simulink model "airTrackHangingMass"  (R2021a)
settings: Solver=VariableStepAuto  StartTime=0.0  StopTime=30  FixedStep=0.02  MaxStep=0.002  RelTol=1e-6  EnableMultiTasking=on
PostLoadFcn:
  | disp('default settings')
  | 
  | % Default starting positions
  | x0_cart1 = -0.2
  | x0_cart2 = 0.8
  | x0_gate1 = -0.4
  | x0_gate2 = 0.4
  | 
  | % How much damping the carts feel
  | dampingCoef = 0.01 % N/(m/s)
  | 
  | % Hanger damping
  | pulleyDamping = 0;
  | 
  | % Max measurement noise for the gates
  | noise_max = 0.01 % seconds
  | 
  | % How many time steps to show in the history
  | nHistory = 4
  | 
  | % Based on the provided STLs
  | cart_length = 0.15
  | 
  | subsystems = find_system(gcs,'BlockType','SubSystem');
  | p = Simulink.Mask.get(subsystems{1});
  | p.Parameters(1).Value = '-0.8';
  | p.Parameters(2).Value = '0';
  | p.Parameters(3).Value = '-0.4';
  | p.Parameters(4).Value = '0.4';
  | p.Parameters(5).Value = '0';
  | p.Parameters(6).Value = '0';
  | p.Parameters(7).Value = '20';
undefined symbols (not defined in the file): Push, X, x, Y, Z
libraries: sm_lib x73, simulink x12, nesl_utility x7
(part 3 of 3)

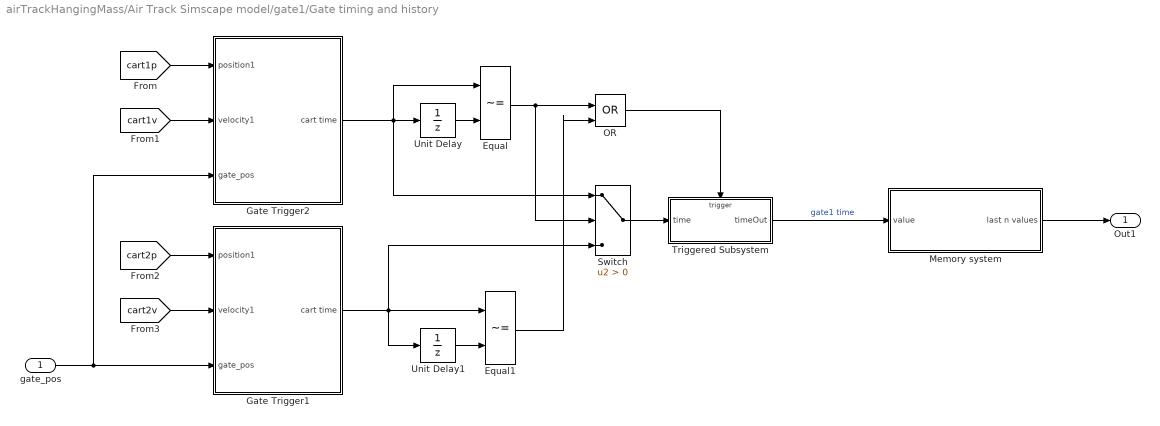
== system airTrackHangingMass/Air Track Simscape model/gate1/Gate timing and history ==
  gate_pos : Inport
  Equal : RelationalOperator  Operator=~=  OutDataTypeStr=boolean  RndMeth=Simplest
  Equal1 : RelationalOperator  Operator=~=  OutDataTypeStr=boolean  RndMeth=Simplest
  Gate Trigger1 : Subsystem
  Gate Trigger2 : Subsystem
  Memory system : Subsystem
  OR : Logic  Operator=OR  IconShape=distinctive  AllPortsSameDT=off  OutDataTypeStr=boolean
  Switch : Switch  Criteria=u2 > Threshold
  Triggered Subsystem : Subsystem  TreatAsAtomicUnit=on
  Unit Delay : UnitDelay  SampleTime=-1  HasFrameUpgradeWarning=on
  Unit Delay1 : UnitDelay  SampleTime=-1  HasFrameUpgradeWarning=on
  Out1 : Outport
  wires:
  Gate Trigger1/1(cart time) -> Switch/3, Equal1/1, Unit Delay1/1
  gate_pos/1 -> Gate Trigger2/3(gate_pos), Gate Trigger1/3(gate_pos)
  OR/1 -> Triggered Subsystem/Trigger
  [cart2p] -> Gate Trigger1/1(position1)
  Equal/1 -> Switch/2, OR/1
  [cart1v] -> Gate Trigger2/2(velocity1)
  Triggered Subsystem/1(timeOut) -> Memory system/1(value)  "gate1 time"
  [cart2v] -> Gate Trigger1/2(velocity1)
  Unit Delay/1 -> Equal/2
  Gate Trigger2/1(cart time) -> Switch/1, Equal/1, Unit Delay/1
  Equal1/1 -> OR/2
  Unit Delay1/1 -> Equal1/2
  [cart1p] -> Gate Trigger2/1(position1)
  Switch/1 -> Triggered Subsystem/1(time)
  Memory system/1(last n values) -> Out1/1

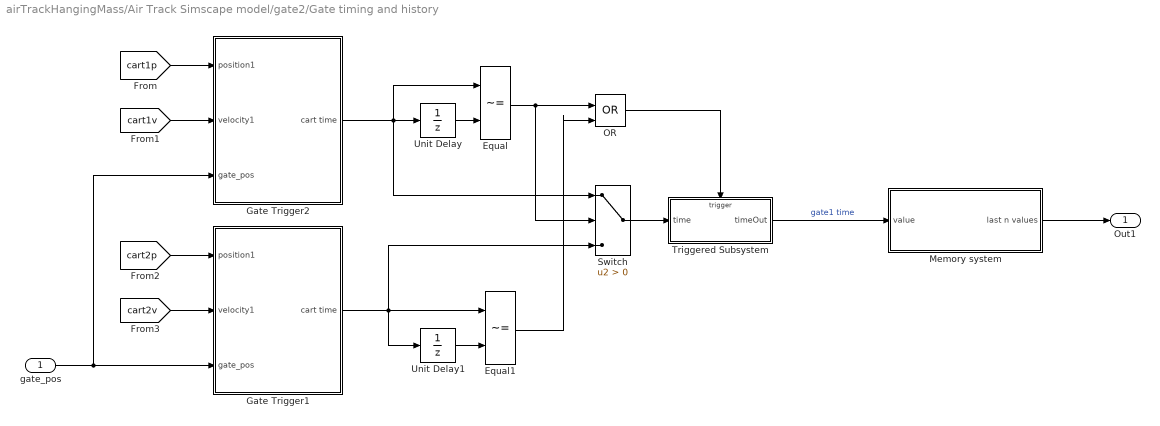
== system airTrackHangingMass/Air Track Simscape model/gate2/Gate timing and history ==
  gate_pos : Inport
  Equal : RelationalOperator  Operator=~=  OutDataTypeStr=boolean  RndMeth=Simplest
  Equal1 : RelationalOperator  Operator=~=  OutDataTypeStr=boolean  RndMeth=Simplest
  Gate Trigger1 : Subsystem
  Gate Trigger2 : Subsystem
  Memory system : Subsystem
  OR : Logic  Operator=OR  IconShape=distinctive  AllPortsSameDT=off  OutDataTypeStr=boolean
  Switch : Switch  Criteria=u2 > Threshold
  Triggered Subsystem : Subsystem  TreatAsAtomicUnit=on
  Unit Delay : UnitDelay  SampleTime=-1  HasFrameUpgradeWarning=on
  Unit Delay1 : UnitDelay  SampleTime=-1  HasFrameUpgradeWarning=on
  Out1 : Outport
  wires:
  Gate Trigger1/1(cart time) -> Switch/3, Equal1/1, Unit Delay1/1
  gate_pos/1 -> Gate Trigger2/3(gate_pos), Gate Trigger1/3(gate_pos)
  OR/1 -> Triggered Subsystem/Trigger
  [cart2p] -> Gate Trigger1/1(position1)
  Equal/1 -> Switch/2, OR/1
  [cart1v] -> Gate Trigger2/2(velocity1)
  Triggered Subsystem/1(timeOut) -> Memory system/1(value)  "gate1 time"
  [cart2v] -> Gate Trigger1/2(velocity1)
  Unit Delay/1 -> Equal/2
  Gate Trigger2/1(cart time) -> Switch/1, Equal/1, Unit Delay/1
  Equal1/1 -> OR/2
  Unit Delay1/1 -> Equal1/2
  [cart1p] -> Gate Trigger2/1(position1)
  Switch/1 -> Triggered Subsystem/1(time)
  Memory system/1(last n values) -> Out1/1

== system airTrackHangingMass/Air Track Simscape model/Cart1/short pulse/Triggered Subsystem ==
  In1 : Inport
  Trigger : TriggerPort  VariantControl=Variant
  Out1 : Outport
  wires:
  In1/1 -> Out1/1

== system airTrackHangingMass/Air Track Simscape model/Cart1/short pulse/Triggered Subsystem1 ==
  In1 : Inport
  Trigger : TriggerPort  VariantControl=Variant
  Out1 : Outport
  wires:
  In1/1 -> Out1/1

== system airTrackHangingMass/Air Track Simscape model/Cart2/short pulse2/Triggered Subsystem ==
  In1 : Inport
  Trigger : TriggerPort  VariantControl=Variant
  Out1 : Outport
  wires:
  In1/1 -> Out1/1

== system airTrackHangingMass/Air Track Simscape model/Cart2/short pulse2/Triggered Subsystem1 ==
  In1 : Inport
  Trigger : TriggerPort  VariantControl=Variant
  Out1 : Outport
  wires:
  In1/1 -> Out1/1

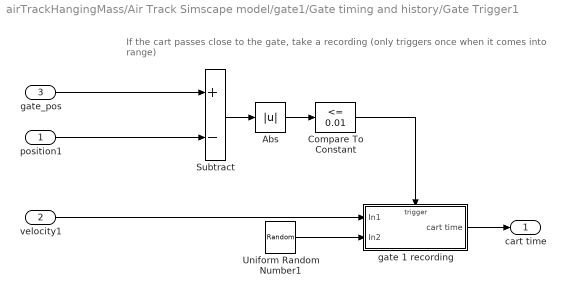
== system airTrackHangingMass/Air Track Simscape model/gate1/Gate timing and history/Gate Trigger1 ==
  note: If the cart passes close to the gate, take a recording
      | (only triggers once when it comes into range)
  position1 : Inport
  velocity1 : Inport  Port=2
  gate_pos : Inport  Port=3
  Abs : Abs
  Compare To Constant : simulink/Logic and Bit Operations/Compare To Constant  relop=<=  const=0.01  OutDataTypeStr=boolean
  Subtract : Sum  Inputs=+-
  Uniform Random Number1 : UniformRandomNumber  Minimum=-noise_max/2  Maximum=noise_max/2  SampleTime=0.1
  gate 1 recording : Subsystem  TreatAsAtomicUnit=on
  cart time : Outport
  wires:
  position1/1 -> Subtract/2
  velocity1/1 -> gate 1 recording/1(In1)
  gate 1 recording/1(cart time) -> cart time/1
  Abs/1 -> Compare To Constant/1
  Subtract/1 -> Abs/1
  Compare To Constant/1 -> gate 1 recording/Trigger
  Uniform Random Number1/1 -> gate 1 recording/2(In2)
  gate_pos/1 -> Subtract/1

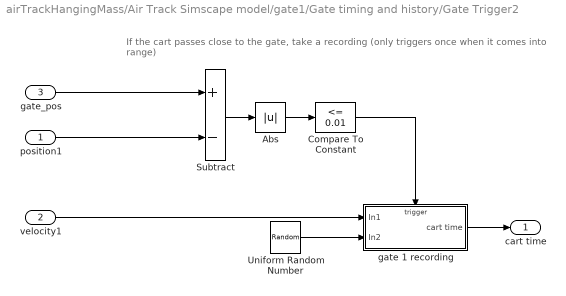
== system airTrackHangingMass/Air Track Simscape model/gate1/Gate timing and history/Gate Trigger2 ==
  note: If the cart passes close to the gate, take a recording
      | (only triggers once when it comes into range)
  position1 : Inport
  velocity1 : Inport  Port=2
  gate_pos : Inport  Port=3
  Abs : Abs
  Compare To Constant : simulink/Logic and Bit Operations/Compare To Constant  relop=<=  const=0.01  OutDataTypeStr=boolean
  Subtract : Sum  Inputs=+-
  Uniform Random Number : UniformRandomNumber  Minimum=-noise_max/2  Maximum=noise_max/2  SampleTime=0.1
  gate 1 recording : Subsystem  TreatAsAtomicUnit=on
  cart time : Outport
  wires:
  position1/1 -> Subtract/2
  velocity1/1 -> gate 1 recording/1(In1)
  gate 1 recording/1(cart time) -> cart time/1
  Abs/1 -> Compare To Constant/1
  Subtract/1 -> Abs/1
  Compare To Constant/1 -> gate 1 recording/Trigger
  Uniform Random Number/1 -> gate 1 recording/2(In2)
  gate_pos/1 -> Subtract/1

== system airTrackHangingMass/Air Track Simscape model/gate1/Gate timing and history/Memory system ==
  value : Inport
  Assignment : Assignment  DiagnosticForDimensions=Warning  IndexOptions=Index vector (dialog)  Indices=1  OutputSizes=1
  Equal : RelationalOperator  Operator=~=  OutDataTypeStr=boolean  RndMeth=Simplest
  Triggered Subsystem : Subsystem  TreatAsAtomicUnit=on
  Unit Delay : UnitDelay  InitialCondition=zeros(nHistory,1)  SampleTime=-1  HasFrameUpgradeWarning=on
  Unit Delay1 : UnitDelay  SampleTime=-1  HasFrameUpgradeWarning=on
  last n values : Outport
  wires:
  Unit Delay/1 -> Triggered Subsystem/1(In1)
  Assignment/1 -> Unit Delay/1, last n values/1
  value/1 -> Equal/1, Unit Delay1/1, Assignment/2
  Triggered Subsystem/1(Out1) -> Assignment/1
  Equal/1 -> Triggered Subsystem/Trigger
  Unit Delay1/1 -> Equal/2

== system airTrackHangingMass/Air Track Simscape model/gate1/Gate timing and history/Triggered Subsystem ==
  time : Inport
  Trigger : TriggerPort  VariantControl=Variant
  timeOut : Outport
  wires:
  time/1 -> timeOut/1

== system airTrackHangingMass/Air Track Simscape model/gate2/Gate timing and history/Gate Trigger1 ==
  note: If the cart passes close to the gate, take a recording
      | (only triggers once when it comes into range)
  position1 : Inport
  velocity1 : Inport  Port=2
  gate_pos : Inport  Port=3
  Abs : Abs
  Compare To Constant : simulink/Logic and Bit Operations/Compare To Constant  relop=<=  const=0.01  OutDataTypeStr=boolean
  Subtract : Sum  Inputs=+-
  Uniform Random Number1 : UniformRandomNumber  Minimum=-noise_max/2  Maximum=noise_max/2  SampleTime=0.1
  gate 1 recording : Subsystem  TreatAsAtomicUnit=on
  cart time : Outport
  wires:
  position1/1 -> Subtract/2
  velocity1/1 -> gate 1 recording/1(In1)
  gate 1 recording/1(cart time) -> cart time/1
  Abs/1 -> Compare To Constant/1
  Subtract/1 -> Abs/1
  Compare To Constant/1 -> gate 1 recording/Trigger
  Uniform Random Number1/1 -> gate 1 recording/2(In2)
  gate_pos/1 -> Subtract/1

== system airTrackHangingMass/Air Track Simscape model/gate2/Gate timing and history/Gate Trigger2 ==
  note: If the cart passes close to the gate, take a recording
      | (only triggers once when it comes into range)
  position1 : Inport
  velocity1 : Inport  Port=2
  gate_pos : Inport  Port=3
  Abs : Abs
  Compare To Constant : simulink/Logic and Bit Operations/Compare To Constant  relop=<=  const=0.01  OutDataTypeStr=boolean
  Subtract : Sum  Inputs=+-
  Uniform Random Number1 : UniformRandomNumber  Minimum=-noise_max/2  Maximum=noise_max/2  SampleTime=0.1
  gate 1 recording : Subsystem  TreatAsAtomicUnit=on
  cart time : Outport
  wires:
  position1/1 -> Subtract/2
  velocity1/1 -> gate 1 recording/1(In1)
  gate 1 recording/1(cart time) -> cart time/1
  Abs/1 -> Compare To Constant/1
  Subtract/1 -> Abs/1
  Compare To Constant/1 -> gate 1 recording/Trigger
  Uniform Random Number1/1 -> gate 1 recording/2(In2)
  gate_pos/1 -> Subtract/1

== system airTrackHangingMass/Air Track Simscape model/gate2/Gate timing and history/Memory system ==
  value : Inport
  Assignment : Assignment  DiagnosticForDimensions=Warning  IndexOptions=Index vector (dialog)  Indices=1  OutputSizes=1
  Equal : RelationalOperator  Operator=~=  OutDataTypeStr=boolean  RndMeth=Simplest
  Triggered Subsystem : Subsystem  TreatAsAtomicUnit=on
  Unit Delay : UnitDelay  InitialCondition=zeros(nHistory,1)  SampleTime=-1  HasFrameUpgradeWarning=on
  Unit Delay1 : UnitDelay  SampleTime=-1  HasFrameUpgradeWarning=on
  last n values : Outport
  wires:
  Unit Delay/1 -> Triggered Subsystem/1(In1)
  Assignment/1 -> Unit Delay/1, last n values/1
  value/1 -> Equal/1, Unit Delay1/1, Assignment/2
  Triggered Subsystem/1(Out1) -> Assignment/1
  Equal/1 -> Triggered Subsystem/Trigger
  Unit Delay1/1 -> Equal/2

== system airTrackHangingMass/Air Track Simscape model/gate2/Gate timing and history/Triggered Subsystem ==
  time : Inport
  Trigger : TriggerPort  VariantControl=Variant
  timeOut : Outport
  wires:
  time/1 -> timeOut/1

== system airTrackHangingMass/Air Track Simscape model/gate1/Gate timing and history/Gate Trigger1/gate 1 recording ==
  In1 : Inport
  In2 : Inport  Port=2
  Trigger : TriggerPort  VariantControl=Variant
  Abs : Abs
  Divide : Product  Inputs=*/
  Sum : Sum  Inputs=|++
  cart length (meters) : Constant  Value=cart_length
  cart time : Outport
  wires:
  In2/1 -> Sum/2
  Sum/1 -> cart time/1
  Abs/1 -> Sum/1
  Divide/1 -> Abs/1
  In1/1 -> Divide/2
  cart length (meters)/1 -> Divide/1

== system airTrackHangingMass/Air Track Simscape model/gate1/Gate timing and history/Gate Trigger2/gate 1 recording ==
  In1 : Inport
  In2 : Inport  Port=2
  Trigger : TriggerPort  VariantControl=Variant
  Abs : Abs
  Divide : Product  Inputs=*/
  Sum : Sum  Inputs=|++
  cart length (meters) : Constant  Value=cart_length
  cart time : Outport
  wires:
  In2/1 -> Sum/2
  Sum/1 -> cart time/1
  Abs/1 -> Sum/1
  Divide/1 -> Abs/1
  In1/1 -> Divide/2
  cart length (meters)/1 -> Divide/1

== system airTrackHangingMass/Air Track Simscape model/gate1/Gate timing and history/Memory system/Triggered Subsystem ==
  In1 : Inport
  Trigger : TriggerPort  VariantControl=Variant
  For Iterator Subsystem : Subsystem  TreatAsAtomicUnit=on
  Out1 : Outport
  wires:
  In1/1 -> For Iterator Subsystem/1(In1)
  For Iterator Subsystem/1(Out1) -> Out1/1

== system airTrackHangingMass/Air Track Simscape model/gate2/Gate timing and history/Gate Trigger1/gate 1 recording ==
  In1 : Inport
  In2 : Inport  Port=2
  Trigger : TriggerPort  VariantControl=Variant
  Abs : Abs
  Divide : Product  Inputs=*/
  Sum : Sum  Inputs=|++
  cart length (meters) : Constant  Value=cart_length
  cart time : Outport
  wires:
  In2/1 -> Sum/2
  Sum/1 -> cart time/1
  Abs/1 -> Sum/1
  Divide/1 -> Abs/1
  In1/1 -> Divide/2
  cart length (meters)/1 -> Divide/1

== system airTrackHangingMass/Air Track Simscape model/gate2/Gate timing and history/Gate Trigger2/gate 1 recording ==
  In1 : Inport
  In2 : Inport  Port=2
  Trigger : TriggerPort  VariantControl=Variant
  Abs : Abs
  Divide : Product  Inputs=*/
  Sum : Sum  Inputs=|++
  cart length (meters) : Constant  Value=cart_length
  cart time : Outport
  wires:
  In2/1 -> Sum/2
  Sum/1 -> cart time/1
  Abs/1 -> Sum/1
  Divide/1 -> Abs/1
  In1/1 -> Divide/2
  cart length (meters)/1 -> Divide/1

== system airTrackHangingMass/Air Track Simscape model/gate2/Gate timing and history/Memory system/Triggered Subsystem ==
  In1 : Inport
  Trigger : TriggerPort  VariantControl=Variant
  For Iterator Subsystem : Subsystem  TreatAsAtomicUnit=on
  Out1 : Outport
  wires:
  In1/1 -> For Iterator Subsystem/1(In1)
  For Iterator Subsystem/1(Out1) -> Out1/1

== system airTrackHangingMass/Air Track Simscape model/gate1/Gate timing and history/Memory system/Triggered Subsystem/For Iterator Subsystem ==
  In1 : Inport
  Assignment : Assignment  DiagnosticForDimensions=Warning  IndexOptions=Index vector (port)  Indices=1  OutputSizes=1
  Bias : Bias  Bias=1
  For Iterator : ForIterator  IterationLimit=nHistory-1
  Selector : Selector  InputPortWidth=nHistory  IndexOptions=Index vector (port)  Indices=[1 3]  OutputSizes=1
  Out1 : Outport
  wires:
  For Iterator/1 -> Bias/1, Selector/2
  Assignment/1 -> Out1/1
  In1/1 -> Assignment/1, Selector/1
  Bias/1 -> Assignment/3
  Selector/1 -> Assignment/2

== system airTrackHangingMass/Air Track Simscape model/gate2/Gate timing and history/Memory system/Triggered Subsystem/For Iterator Subsystem ==
  In1 : Inport
  Assignment : Assignment  DiagnosticForDimensions=Warning  IndexOptions=Index vector (port)  Indices=1  OutputSizes=1
  Bias : Bias  Bias=1
  For Iterator : ForIterator  IterationLimit=nHistory-1
  Selector : Selector  InputPortWidth=nHistory  IndexOptions=Index vector (port)  Indices=[1 3]  OutputSizes=1
  Out1 : Outport
  wires:
  For Iterator/1 -> Bias/1, Selector/2
  Assignment/1 -> Out1/1
  In1/1 -> Assignment/1, Selector/1
  Bias/1 -> Assignment/3
  Selector/1 -> Assignment/2
